simulink model "model"  (R2024a)
settings: Solver=ode15s  StartTime=0.0  StopTime=0.25  FixedStep=1e-4  RelTol=1e-3
undefined symbols (not defined in the file): data, data_SL_Info, effort, effort_SL_Info, name, name_SL_Info, position, position_SL_Info, velocity, velocity_SL_Info, X, Y, Z
libraries: sm_lib x45, nesl_utility x14, ros2lib x6
(part 2 of 2)

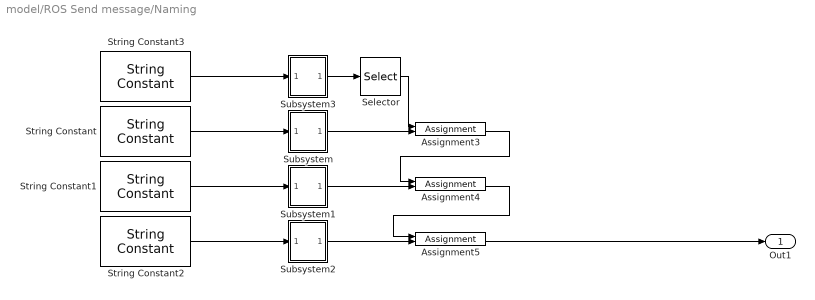
== system model/ROS Send message/Naming ==
  Assignment3 : Assignment  DiagnosticForDimensions=Warning  IndexOptions=Index vector (dialog)  Indices=1  OutputSizes=1
  Assignment4 : Assignment  DiagnosticForDimensions=Warning  IndexOptions=Index vector (dialog)  Indices=2  OutputSizes=1
  Assignment5 : Assignment  DiagnosticForDimensions=Warning  IndexOptions=Index vector (dialog)  Indices=3  OutputSizes=1
  Selector : Selector  InputPortWidth=1  IndexOptions=Index vector (dialog)  Indices=ones([1,16])  OutputSizes=1
  String Constant : StringConstant  String="\"joint1_rev_a\""
  String Constant1 : StringConstant  String="\"joint2_prism_h\""
  String Constant2 : StringConstant  String="\"joint3_prism_l\""
  String Constant3 : StringConstant  String="\"\""
  Subsystem : Subsystem
  Subsystem1 : Subsystem
  Subsystem2 : Subsystem
  Subsystem3 : Subsystem
  Out1 : Outport
  wires:
  String Constant/1 -> Subsystem/1(In1)
  Assignment4/1 -> Assignment5/1
  String Constant2/1 -> Subsystem2/1(In1)
  Subsystem/1(Out1) -> Assignment3/2
  Assignment3/1 -> Assignment4/1
  Selector/1 -> Assignment3/1
  String Constant3/1 -> Subsystem3/1(In1)
  Subsystem1/1(Out1) -> Assignment4/2
  Subsystem3/1(Out1) -> Selector/1
  String Constant1/1 -> Subsystem1/1(In1)
  Subsystem2/1(Out1) -> Assignment5/2
  Assignment5/1 -> Out1/1

== system model/ROS Send message/Naming/Subsystem ==
  In1 : Inport
  Bus Assignment1 : BusAssignment  AssignedSignals=data,data_SL_Info.CurrentLength
  Constant3 : Constant  Value=0  OutDataTypeStr=Bus: SL_Bus_std_msgs_String
  Constant4 : Constant  Value=128  OutDataTypeStr=uint32
  String to ASCII : StringToASCII  OutputVectorSize=128
  Out1 : Outport
  wires:
  String to ASCII/1 -> Bus Assignment1/2
  Constant4/1 -> Bus Assignment1/3
  Constant3/1 -> Bus Assignment1/1
  Bus Assignment1/1 -> Out1/1
  In1/1 -> String to ASCII/1

== system model/ROS Send message/Naming/Subsystem1 ==
  In1 : Inport
  Bus Assignment1 : BusAssignment  AssignedSignals=data,data_SL_Info.CurrentLength
  Constant3 : Constant  Value=0  OutDataTypeStr=Bus: SL_Bus_std_msgs_String
  Constant4 : Constant  Value=128  OutDataTypeStr=uint32
  String to ASCII : StringToASCII  OutputVectorSize=128
  Out1 : Outport
  wires:
  String to ASCII/1 -> Bus Assignment1/2
  Constant4/1 -> Bus Assignment1/3
  Constant3/1 -> Bus Assignment1/1
  Bus Assignment1/1 -> Out1/1
  In1/1 -> String to ASCII/1

== system model/ROS Send message/Naming/Subsystem2 ==
  In1 : Inport
  Bus Assignment1 : BusAssignment  AssignedSignals=data,data_SL_Info.CurrentLength
  Constant3 : Constant  Value=0  OutDataTypeStr=Bus: SL_Bus_std_msgs_String
  Constant4 : Constant  Value=128  OutDataTypeStr=uint32
  String to ASCII : StringToASCII  OutputVectorSize=128
  Out1 : Outport
  wires:
  String to ASCII/1 -> Bus Assignment1/2
  Constant4/1 -> Bus Assignment1/3
  Constant3/1 -> Bus Assignment1/1
  Bus Assignment1/1 -> Out1/1
  In1/1 -> String to ASCII/1

== system model/ROS Send message/Naming/Subsystem3 ==
  In1 : Inport
  Bus Assignment1 : BusAssignment  AssignedSignals=data,data_SL_Info.CurrentLength
  Constant3 : Constant  Value=0  OutDataTypeStr=Bus: SL_Bus_std_msgs_String
  Constant4 : Constant  Value=128  OutDataTypeStr=uint32
  String to ASCII : StringToASCII  OutputVectorSize=128
  Out1 : Outport
  wires:
  String to ASCII/1 -> Bus Assignment1/2
  Constant4/1 -> Bus Assignment1/3
  Constant3/1 -> Bus Assignment1/1
  Bus Assignment1/1 -> Out1/1
  In1/1 -> String to ASCII/1
